simulink library "Simulink_Library_Example_Lib"  (R2021b)
settings: Solver=VariableStepAuto  StartTime=0.0  StopTime=10.0  RelTol=1e-3
settings Model: Creator=waleed.elshemy  LastModifiedBy=waleed.elshemy

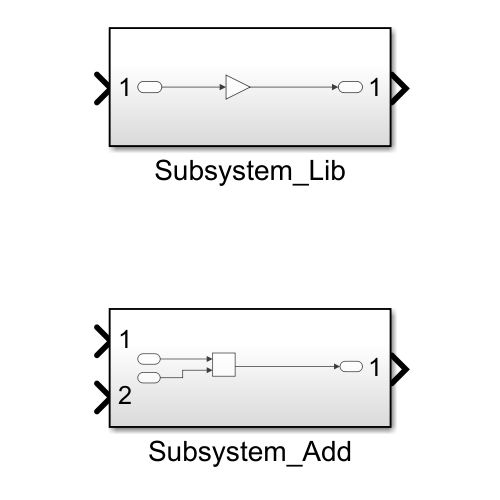
[thumbnail: Simulink's stored preview of the top-level diagram]
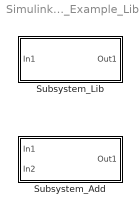
== system Simulink_Library_Example_Lib ==
  Subsystem_Add : Subsystem
  Subsystem_Lib : Subsystem

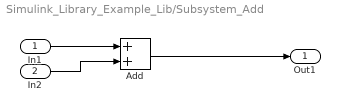
== system Simulink_Library_Example_Lib/Subsystem_Add ==
  In1 : Inport
  In2 : Inport  Port=2
  Add : Sum
  Out1 : Outport
  wires:
  In1/1 -> Add/1
  In2/1 -> Add/2
  Add/1 -> Out1/1

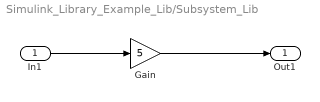
== system Simulink_Library_Example_Lib/Subsystem_Lib ==
  In1 : Inport
  Gain : Gain  Gain=5
  Out1 : Outport
  wires:
  In1/1 -> Gain/1
  Gain/1 -> Out1/1
